simulink model "Demo2"  (R2025b)
settings: Solver=VariableStepAuto  StartTime=0.0  StopTime=Inf  RelTol=1e-3
settings Model: Creator=Soochan Kim  LastModifiedBy=Soochan Kim
settings OptimizationCC: BlockReduction=off  ConditionallyExecuteInputs=off  DefaultParameterBehavior=Inlined
settings DebuggingCC: AlgebraicLoopMsg=error
settings HardwareCC: ProdBitPerPointer=32.0  ProdBitPerSizeT=32.0  ProdBitPerPtrDiffT=32.0  ProdLargestAtomicFloat=None  ProdIntDivRoundTo=Undefined  ProdEndianess=Unspecified  ProdWordSize=32.0  ProdHWDeviceType=ASIC/FPGA->ASIC/FPGA  TargetBitPerPointer=64.0  TargetBitPerSizeT=64.0  TargetBitPerPtrDiffT=64.0  TargetLongLongMode=on  TargetIntDivRoundTo=Zero  TargetEndianess=LittleEndian  TargetWordSize=64.0  TargetHWDeviceType=Custom Processor->MATLAB Host Computer  ProdEqTarget=off

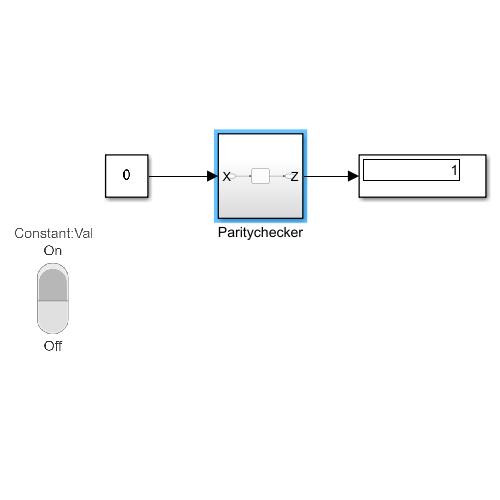
[thumbnail: Simulink's stored preview of the top-level diagram]
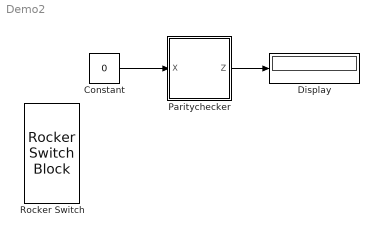
== system Demo2 ==
  Constant : Constant  Value=0  OutDataTypeStr=boolean
  Display : Display
  Paritychecker : Subsystem
  Rocker Switch : RockerSwitchBlock
  wires:
  Constant/1 -> Paritychecker/1(X)
  Paritychecker/1(Z) -> Display/1

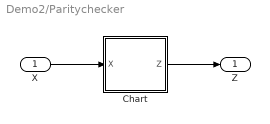
== system Demo2/Paritychecker ==
  X : Inport
  Chart : Stateflow chart  TreatAsAtomicUnit=on
  Z : Outport
  wires:
  Chart/1(Z) -> Z/1
  X/1 -> Chart/1(X)

== stateflow chart Demo2/Paritychecker/Chart ==
  settings: updateMethod=DISCRETE  sampleTime=1  stateMachineType=MOORE_MACHINE  executeAtInitialization=1  initializeOutput=1
  state S0
    Z = false;
  state S1
    Z = true;
  (default) -> S0
  S0 -> S1 : [X==1]
  S1 -> S0 : [X==1]
  data: Z output; X input
